simulink model "simulink_ej3"  (R2021a)
settings: Solver=FixedStepAuto  StartTime=0.0  StopTime=5  FixedStep=0.001  RelTol=1e-3
libraries: roblocks x1
settings Model: Creator=omsma  LastModifiedBy=omsma

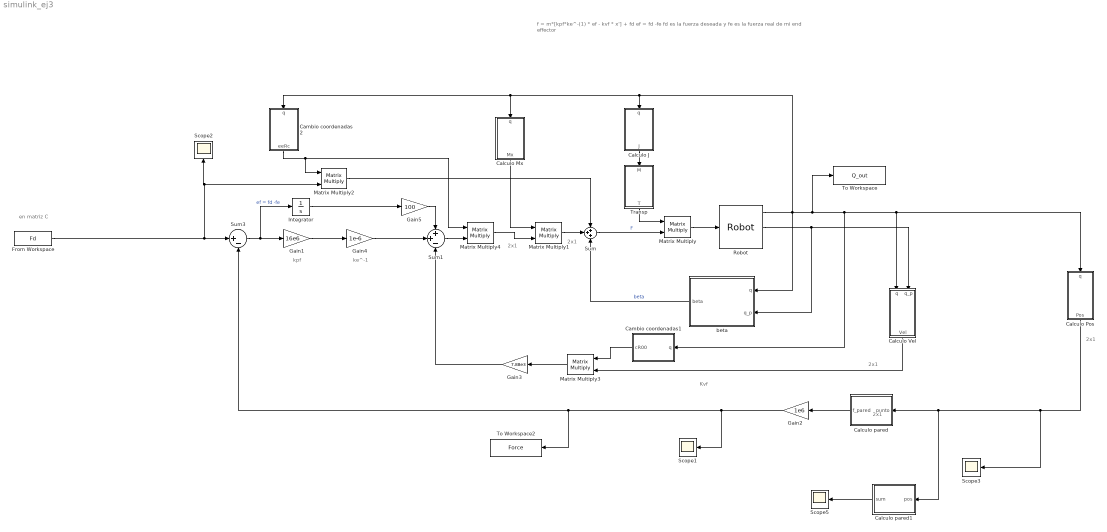
== system simulink_ej3 ==
  note: en matriz C
  note: 2x1
  note: ke^-1
  note: 2x1
  note: 2x1
  note: 2x1
  note: Kvf
  note: 2x1
  note: f = m*[kpf*ke^-(1) * ef - kvf * x'] + fd
      |
      | ef = fd -fe
      | fd es la fuerza deseada y fe es la fuerza real de mi end effector
  note: kpf
  Calculo J : MATLAB Function  TreatAsAtomicUnit=on
  Calculo Mx : MATLAB Function  TreatAsAtomicUnit=on
  Calculo Pos : MATLAB Function  TreatAsAtomicUnit=on
  Calculo Vel : MATLAB Function  TreatAsAtomicUnit=on
  Calculo pared : MATLAB Function  TreatAsAtomicUnit=on
  Calculo pared1 : MATLAB Function  TreatAsAtomicUnit=on
  Cambio coordenadas1 : MATLAB Function  TreatAsAtomicUnit=on
  Cambio coordenadas2 : MATLAB Function  TreatAsAtomicUnit=on
  From Workspace : FromWorkspace  VariableName=Fd
  Gain1 : Gain  Gain=16e6
  Gain2 : Gain  Gain=1e6
  Gain3 : Gain  Gain=7.88e3
  Gain4 : Gain  Gain=1e-6
  Gain5 : Gain  Gain=100
  Integrator : Integrator
  Matrix Multiply{,1..4} (5 alike) : Product  Multiplication=Matrix(*)
  Robot : roblocks/Arm/Robot  robot=rob  q0=[1.9291, -1.1437]
      link override Integrator1: InitialCondition=q_inicial
  Scope{1..3,5} (4 alike) : Scope
  Sum : Sum  Inputs=+++
  Sum1 : Sum  Inputs=++-
  Sum3 : Sum  Inputs=|+-
  To Workspace : ToWorkspace  VariableName=Q_out  SampleTime=-1
      settings: Save2DSignal=2-D array (concatenate along first dimension)
  To Workspace2 : ToWorkspace  VariableName=Force  SaveFormat=Timeseries  SampleTime=-1
  Transp : MATLAB Function  TreatAsAtomicUnit=on
  beta : MATLAB Function  TreatAsAtomicUnit=on
  wires:
  Calculo Pos/1(Pos) -> Scope3/1, Calculo pared1/1(pos), Calculo pared/1(punto)
  Gain5/1 -> Sum1/1
  Cambio coordenadas1/1(cR00) -> Matrix Multiply3/1
  Sum3/1 -> Integrator/1, Gain1/1  "ef = fd -fe"
  beta/1(beta) -> Sum/3  "beta"
  Matrix Multiply/1 -> Robot/1
  Gain4/1 -> Sum1/2
  Gain2/1 -> Scope1/1, To Workspace2/1, Sum3/2
  Integrator/1 -> Gain5/1
  Gain1/1 -> Gain4/1
  Matrix Multiply3/1 -> Gain3/1
  Calculo pared/1(f_pared) -> Gain2/1
  Robot/1 -> beta/1(q), Calculo J/1(q), Cambio coordenadas2/1(q), Calculo Mx/1(q), Cambio coordenadas1/1(q), Calculo Pos/1(q), Calculo Vel/1(q), To Workspace/1
  Robot/2 -> Calculo Vel/2(q_p), beta/2(q_p)
  Gain3/1 -> Sum1/3
  Sum/1 -> Matrix Multiply/2  "F"
  Calculo J/1(J) -> Transp/1(M)
  Calculo Vel/1(Vel) -> Matrix Multiply3/2
  Transp/1(T) -> Matrix Multiply/1
  Matrix Multiply1/1 -> Sum/2
  Calculo Mx/1(Mx) -> Matrix Multiply1/1
  From Workspace/1 -> Sum3/1, Matrix Multiply2/2, Scope2/1
  Cambio coordenadas2/1(eeRc) -> Matrix Multiply4/1, Matrix Multiply2/1
  Matrix Multiply2/1 -> Sum/1
  Sum1/1 -> Matrix Multiply4/2
  Matrix Multiply4/1 -> Matrix Multiply1/2
  Calculo pared1/1(sum) -> Scope5/1

== matlab function simulink_ej3/Cambio coordenadas2 ==
  data: q input; eeRc output
function eeRc = eeRc(q)

t1 = q(1);
t2 = q(2);


% ee R c = ee R 00 * 00 R c

eeRc = [cos(t1+t2), sin(t1+t2); -sin(t1+t2), cos(t1+t2)]* [cos(pi/4), -sin(pi/4); sin(pi/4), cos(pi/4)];

== matlab function simulink_ej3/Transp ==
  data: M input; T output
function T = T(M)

T = M';

== matlab function simulink_ej3/beta ==
  data: q input; beta output; q_p input
function beta = beta(q, q_p)
%#codegen
coder.extrinsic('gravload_wrapper');
coder.extrinsic('friction_wrapper');
coder.extrinsic('coriolis_wrapper');

% Preasignaciones
beta = zeros(2,1);
rG = zeros(2,1);
rF = zeros(2,1);
rC = zeros(2,2);
rV = zeros(2,1);


% Llamadas extrínsecas (Simulink ejecutará en MATLAB)
rG = gravload_wrapper([q(1), q(2)]);
rF = friction_wrapper([q_p(1), q_p(2)]);
rC = coriolis_wrapper([q(1), q(2)], [q_p(1), q_p(2)]);

% Cálculos locales
rV = rC * q_p;
beta = rG + rV + rF;
end

== matlab function simulink_ej3/Calculo Mx ==
  data: q input; Mx output
function Mx = Mx(q)

t1 = q(1);
t2 = q(2);

Mx = [(2-cos(t2)^2)/(sin(t2)^2), 0; 0,  1];

== matlab function simulink_ej3/Calculo Pos ==
  data: q input; Pos output
function Pos = Pos(q)

t1 = q(1);
t2 = q(2);

Pos = [cos(t1+t2) + cos(t1); sin(t1+t2) + sin(t1)];

== matlab function simulink_ej3/Calculo Vel ==
  data: q input; Vel output; q_p input
function Vel = Vel(q, q_p)

t1 = q(1);
t2 = q(2);

t1_p = q_p(1);
t2_p = q_p(2);

R = [cos(t1+t2), -sin(t1+t2); 
     sin(t1+t2), cos(t1+t2)];
 
v = [sin(t2)*t1_p; cos(t2)*t1_p];
 
wxp = [0; t1_p+t2_p];

Vel = R*(v + wxp);

== matlab function simulink_ej3/Calculo pared ==
  data: punto input; f_pared output
function f_pared = contacto_pared(punto)
% punto = [x; y] coordenadas del manipulador en la terna base
% Devuelve [delta; 0] en la base de la pared (normal-tangencial)

    % --- Parámetros de la pared ---
    a = 1; b = 1; c = -2;           % Ecuación: x + y - 2 = 0
    n_hat = [a; b] / norm([a b]);   % versor normal a la pared

    % --- Distancia firmada del punto a la pared ---
    d = (a*punto(1) + b*punto(2) + c) / norm([a b]);

    % --- Penetración (solo si hay contacto) ---
    delta = max(0, d);

    % --- Fuerza expresada en la base de la pared ---
    f_pared = [delta; 0];
end

== matlab function simulink_ej3/Cambio coordenadas1 ==
  data: q input; cR00 output
function cR00 = eeRc(q)

t1 = q(1);
t2 = q(2);


% C R 00 = 00 R c

cR00 = [cos(pi/4), sin(pi/4); -sin(pi/4), cos(pi/4)];

== matlab function simulink_ej3/Calculo pared1 ==
  data: pos input; sum output
function sum = calcsum(pos)
    % CALCULO_DISTANCIA_PARED Calcula la distancia del efector final a la pared
    %
    % La pared está definida por: x + y = 2
    % Forma normal: (1/sqrt(2))*x + (1/sqrt(2))*y = 2/sqrt(2) = sqrt(2)
    %
    % Inputs:
    %   pos - Posición del efector final [x; y] o [x, y]
    %
    % Outputs:
    %   d     - Distancia perpendicular a la pared (negativa = penetración)
    %   delta - Magnitud de penetración (0 si no hay contacto, |d| si hay)
    %
    % Ecuación de distancia punto-recta:
    %   d = (x + y - 2) / sqrt(2)
    %   d = n' * [x; y] - d_pared
    %   donde n = [1/sqrt(2); 1/sqrt(2)] y d_pared = sqrt(2)
    
    % Extraer coordenadas
    x = pos(1);
    y = pos(2);
    
    sum = x+y;
end

== matlab function simulink_ej3/Calculo J ==
  data: q input; J output
function J = J(q)

t1 = q(1);
t2 = q(2);

J = [sin(t2), 0; cos(t2)+1, 1];
%J = [0, 0; 0, 0];
